simulink model "hw3_2a_CPG"  (R2013a)
settings: Solver=ode45  StartTime=0.0  StopTime=10.0  RelTol=1e-3
values from neighbouring files (symbols this model uses):
  tx = 1    [hw3_2a_CPGExtensorNeuron.m]
  x0 = 5    [hw3_2a_CPGExtensorNeuron.m]
settings Model: Creator=benshih  LastModifiedBy=benshih

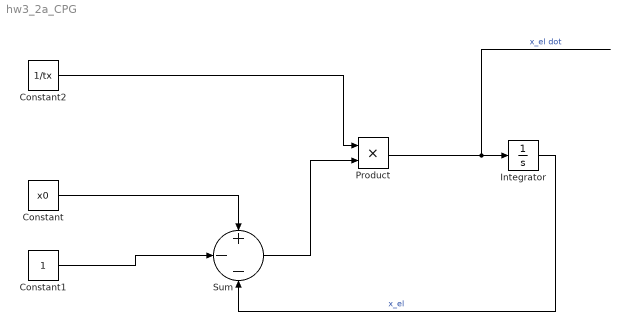
== system hw3_2a_CPG ==
  Constant : Constant  Value=x0
  Constant1 : Constant
  Constant2 : Constant  Value=1/tx
  Integrator : Integrator
  Product : Product
  Sum : Sum  Inputs=+--
  wires:
  Constant2/1 -> Product/1
  Sum/1 -> Product/2
  Product/1 -> Integrator/1  "x_el dot"
  Constant/1 -> Sum/1
  Integrator/1 -> Sum/3  "x_el"
  Constant1/1 -> Sum/2
